simulink model "model_proces_etapa2"  (R2020a)
settings: Solver=VariableStepAuto  StartTime=0.0  StopTime=500  RelTol=1e-3
settings Model: Creator=user  LastModifiedBy=user

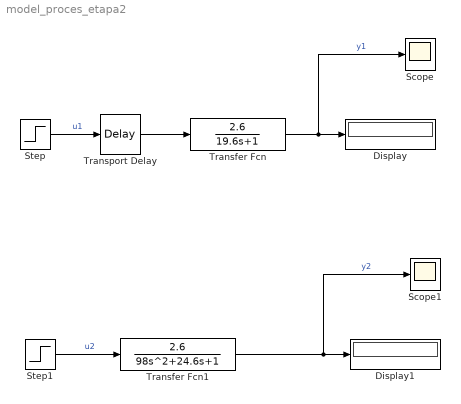
== system model_proces_etapa2 ==
  Display : Display
  Display1 : Display
  Scope : Scope
  Scope1 : Scope
  Step : Step  SampleTime=0
  Step1 : Step  SampleTime=0
  Transfer Fcn : TransferFcn  Numerator=[2.6]  Denominator=[19.6 1]
  Transfer Fcn1 : TransferFcn  Numerator=[2.6]  Denominator=[98 24.6 1]
  Transport Delay : TransportDelay  DelayTime=5
  wires:
  Transfer Fcn1/1 -> Scope1/1, Display1/1  "y2"
  Transport Delay/1 -> Transfer Fcn/1
  Transfer Fcn/1 -> Scope/1, Display/1  "y1"
  Step/1 -> Transport Delay/1  "u1"
  Step1/1 -> Transfer Fcn1/1  "u2"
